simulink model "untitled"  (R2018a)
settings: Solver=VariableStepAuto  StartTime=0.0  StopTime=10.0  RelTol=1e-3
settings Model: Creator=augus  LastModifiedBy=augus

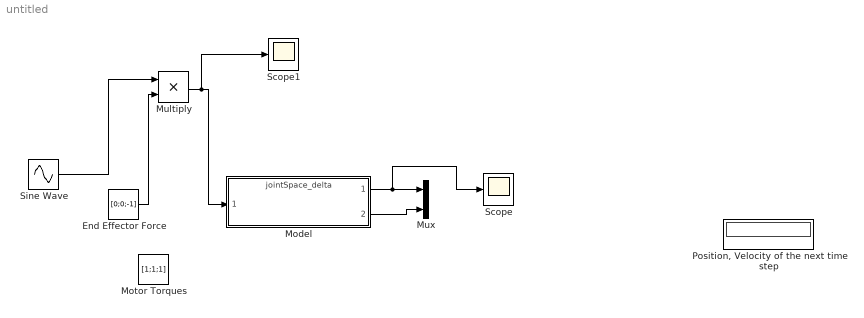
== system untitled ==
  End Effector Force : Constant  Value=[0;0;-1]
  Model : ModelReference  ModelNameDialog=jointSpace_delta  SimulationMode=Normal  ModelReferenceVersion=1.6
  Motor Torques : Constant  Value=[1;1;1]
  Multiply : Product
  Mux : Mux  Inputs=2
  "Position, Velocity of the next time step " : Display
  Scope : Scope
  Scope1 : Scope
  Sine Wave : Sin  SampleTime=0
  wires:
  Multiply/1 -> Scope1/1, Model/1
  Sine Wave/1 -> Multiply/1
  Model/1 -> Scope/1, Mux/1
  End Effector Force/1 -> Multiply/2
  Model/2 -> Mux/2
